simulink model "AllProject"  (R2018b)
settings: Solver=VariableStepAuto  StartTime=0.0  StopTime=10  RelTol=1e-3
values from neighbouring files (symbols this model uses):
  alphaTemperature = (65.5/180)*pi    (= 1.14319066006)    [project.m]
  Ik = 0.38    [project.m]
  Iw = 0.26    [project.m]
  Iz = 1.08    [project.m]
  rk = 0.22    [project.m]
  rw = 0.1    [project.m]
settings Model: Creator=AmirHosein Rostami  LastModifiedBy=AmirHosein Rostami

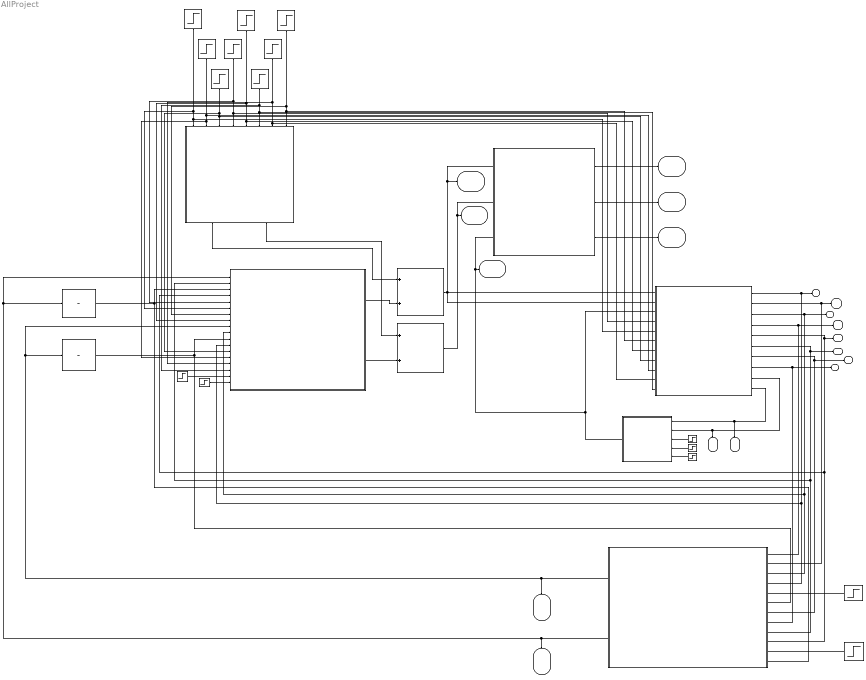
== system AllProject ==
  Add : Sum
  Add1 : Sum
  BallSegway : Subsystem
  Integrator : Integrator
  Integrator1 : Integrator
  LQR : MATLAB Function  TreatAsAtomicUnit=on
  PIController_KP_KI : MATLAB Function  TreatAsAtomicUnit=on
  PIDController : MATLAB Function  TreatAsAtomicUnit=on
  Step : Step  SampleTime=0
  Step1 : Step  SampleTime=0
  Step{10..13} (4 alike) : Step  After=1000  SampleTime=0
  Step2 : Step  After=pi/6  SampleTime=0
  Step{7..9,21} (4 alike) : Step  After=100  SampleTime=0
  Step3 : Step  Time=0  After=0  SampleTime=0
  Step4 : Step  Time=0  After=0  SampleTime=0
  Step5 : Step  After=2.5  SampleTime=0
  Step6 : Step  After=0.2  SampleTime=0
  frictions : MATLAB Function  TreatAsAtomicUnit=on
  torqueConversion2 : MATLAB Function  TreatAsAtomicUnit=on
  TauX : Outport
  TauY : Outport  Port=2
  TauZ : Outport  Port=3
  thetaX : Outport  Port=4
  thetaY : Outport  Port=5
  Vx : Outport  Port=6
  Vy : Outport  Port=7
  xk : Outport  Port=8
  xkDot : Outport  Port=9
  thetaYDot : Outport  Port=10
  yk : Outport  Port=11
  ykDot : Outport  Port=12
  thetaXDot : Outport  Port=13
  Tau1 : Outport  Port=14
  Tau2 : Outport  Port=15
  Tau3 : Outport  Port=16
  thetaZ : Outport  Port=17
  thetaZDot : Outport  Port=18
  wires:
  BallSegway/7("thetaXDot ") -> thetaXDot/1, LQR/7(thetaXDot)
  frictions/1(Uxf) -> Add/1
  frictions/2(Uyf) -> Add1/1
  LQR/1(vx) -> Vx/1, PIController_KP_KI/9(vx), Integrator1/1
  LQR/2(vy) -> Vy/1, PIController_KP_KI/1(vy), Integrator/1
  BallSegway/4("thetaYDot ") -> LQR/1(thetaYDot), thetaYDot/1
  BallSegway/2(thetaY) -> LQR/2(thetaY), thetaY/1
  Integrator/1 -> LQR/12(x5r), PIController_KP_KI/3(x5r)
  Integrator1/1 -> LQR/6(x5p), PIController_KP_KI/11(x5p)
  Add/1 -> BallSegway/2(Taux), TauX/1, torqueConversion2/1(tauX), BallSegway/1(TauY)
  PIDController/1(TauZ) -> BallSegway/3(TauZ), TauZ/1, torqueConversion2/3(tauZ)  "TauZ"
  BallSegway/9(Xz) -> PIDController/2(theta), thetaZ/1  "thetaZ"
  BallSegway/10(XzDot) -> PIDController/1(thetaZDot), thetaZDot/1  "thetaZDot"
  BallSegway/8("thetaX ") -> LQR/8(thetaX), thetaX/1
  Step/1 -> PIDController/3(kdz)
  Step1/1 -> PIDController/4(kpz)
  Step2/1 -> PIDController/5(thetaZDestination)
  BallSegway/1(xk) -> xk/1, LQR/4(xk), PIController_KP_KI/12(xk)
  BallSegway/5(yk) -> yk/1, LQR/10(yk), PIController_KP_KI/4(yk)
  BallSegway/3(xkDot) -> LQR/3(xkDot), PIController_KP_KI/10(xkDot), xkDot/1
  BallSegway/6(ykDot) -> ykDot/1, LQR/9(ykDot), PIController_KP_KI/2(ykDot)
  Step5/1 -> PIController_KP_KI/17(Wn)
  Step6/1 -> PIController_KP_KI/18(kessi)
  Step7/1 -> BallSegway/9(bry), PIController_KP_KI/14(bry), frictions/2(bry)
  Step8/1 -> PIController_KP_KI/13(bx), BallSegway/8(bx), frictions/3(bx)
  Step9/1 -> BallSegway/4(by), frictions/4(by), PIController_KP_KI/5(by)
  Step10/1 -> PIController_KP_KI/8(drx), BallSegway/7(drx), frictions/5(drx)
  Step11/1 -> PIController_KP_KI/16(dry), BallSegway/11(dry), frictions/6(dry)
  Step12/1 -> PIController_KP_KI/15(dx), BallSegway/10(dx), frictions/7(dx)
  Step13/1 -> PIController_KP_KI/7(dy), BallSegway/6(dy), frictions/8(dy)
  Step21/1 -> PIController_KP_KI/6(brx), BallSegway/5(brx), frictions/1(brx)
  PIController_KP_KI/1(uPIx) -> Add/2
  PIController_KP_KI/2(uPIy) -> Add1/2
  torqueConversion2/1(tau1) -> Tau1/1
  torqueConversion2/2(tau2) -> Tau2/1
  torqueConversion2/3(tau3) -> Tau3/1
  Add1/1 -> TauY/1, torqueConversion2/2(tauY)
  Step3/1 -> LQR/11(ykd)
  Step4/1 -> LQR/5(xkd)

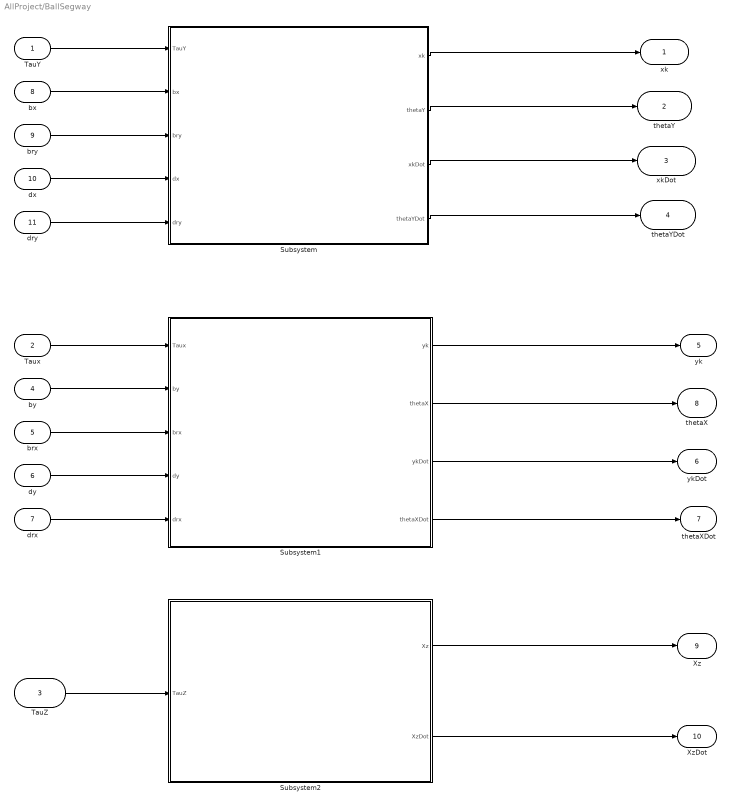
== system AllProject/BallSegway ==
  TauY : Inport
  Taux : Inport  Port=2
  TauZ : Inport  Port=3
  by : Inport  Port=4
  brx : Inport  Port=5
  dy : Inport  Port=6
  drx : Inport  Port=7
  bx : Inport  Port=8
  bry : Inport  Port=9
  dx : Inport  Port=10
  dry : Inport  Port=11
  Subsystem : Subsystem
  Subsystem1 : Subsystem
  Subsystem2 : Subsystem
  xk : Outport
  thetaY : Outport  Port=2
  xkDot : Outport  Port=3
  "thetaYDot " : Outport  Port=4
  yk : Outport  Port=5
  ykDot : Outport  Port=6
  "thetaXDot " : Outport  Port=7
  "thetaX " : Outport  Port=8
  Xz : Outport  Port=9
  XzDot : Outport  Port=10
  wires:
  Subsystem2/1(Xz) -> Xz/1
  TauZ/1 -> Subsystem2/1(TauZ)
  Subsystem2/2(XzDot) -> XzDot/1
  Subsystem/3(xkDot) -> xkDot/1
  Subsystem/4("thetaYDot ") -> "thetaYDot "/1
  Subsystem/1(xk) -> xk/1
  TauY/1 -> Subsystem/1(TauY)
  Taux/1 -> Subsystem1/1(Taux)
  Subsystem1/1(yk) -> yk/1
  Subsystem/2(thetaY) -> thetaY/1
  Subsystem1/4("thetaXDot ") -> "thetaXDot "/1
  Subsystem1/2(thetaX) -> "thetaX "/1
  Subsystem1/3(ykDot) -> ykDot/1
  by/1 -> Subsystem1/2(by)
  brx/1 -> Subsystem1/3(brx)
  dy/1 -> Subsystem1/4(dy)
  drx/1 -> Subsystem1/5(drx)
  bx/1 -> Subsystem/2(bx)
  bry/1 -> Subsystem/3(bry)
  dx/1 -> Subsystem/4(dx)
  dry/1 -> Subsystem/5(dry)

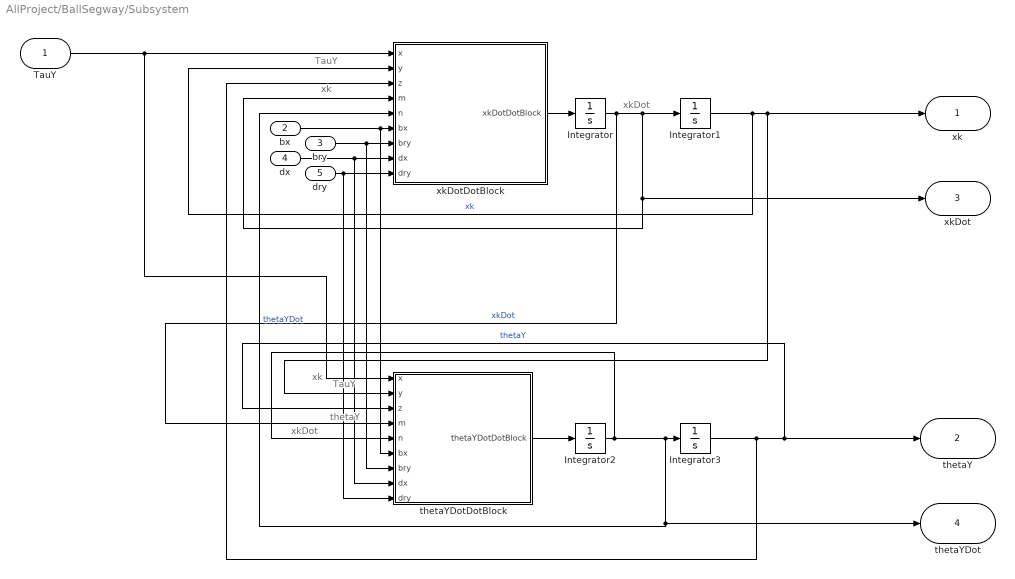
== system AllProject/BallSegway/Subsystem ==
  note: xk
  note: TauY
  note: TauY
  note: xkDot
  note: xk
  note: xkDot
  note: thetaY
  TauY : Inport
  bx : Inport  Port=2
  bry : Inport  Port=3
  dx : Inport  Port=4
  dry : Inport  Port=5
  Integrator : Integrator
  Integrator1 : Integrator
  Integrator2 : Integrator
  Integrator3 : Integrator  InitialCondition=(0.1/180)*pi
  thetaYDotDotBlock : MATLAB Function  TreatAsAtomicUnit=on
  xkDotDotBlock : MATLAB Function  TreatAsAtomicUnit=on
  xk : Outport
  thetaY : Outport  Port=2
  xkDot : Outport  Port=3
  "thetaYDot " : Outport  Port=4
  wires:
  Integrator/1 -> thetaYDotDotBlock/4(m), xkDotDotBlock/4(m), xkDot/1, Integrator1/1  "xkDot"
  Integrator1/1 -> xkDotDotBlock/2(y), thetaYDotDotBlock/2(y), xk/1  "xk"
  Integrator2/1 -> thetaYDotDotBlock/5(n), xkDotDotBlock/5(n), "thetaYDot "/1, Integrator3/1  "thetaYDot"
  xkDotDotBlock/1(xkDotDotBlock) -> Integrator/1
  Integrator3/1 -> xkDotDotBlock/3(z), thetaYDotDotBlock/3(z), thetaY/1  "thetaY"
  TauY/1 -> thetaYDotDotBlock/1(x), xkDotDotBlock/1(x)
  thetaYDotDotBlock/1(thetaYDotDotBlock) -> Integrator2/1
  bx/1 -> thetaYDotDotBlock/6(bx), xkDotDotBlock/6(bx)
  bry/1 -> xkDotDotBlock/7(bry), thetaYDotDotBlock/7(bry)
  dx/1 -> xkDotDotBlock/8(dx), thetaYDotDotBlock/8(dx)
  dry/1 -> xkDotDotBlock/9(dry), thetaYDotDotBlock/9(dry)

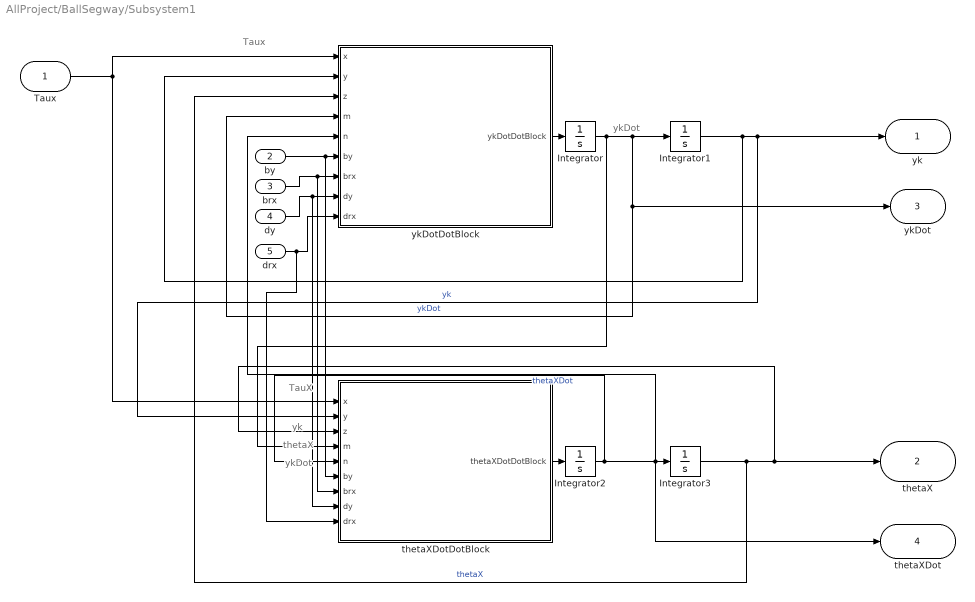
== system AllProject/BallSegway/Subsystem1 ==
  note: yk
  note: Taux
  note: thetaX
  note: ykDot
  note: TauX
  note: ykDot
  Taux : Inport
  by : Inport  Port=2
  brx : Inport  Port=3
  dy : Inport  Port=4
  drx : Inport  Port=5
  Integrator : Integrator
  Integrator1 : Integrator
  Integrator2 : Integrator
  Integrator3 : Integrator  InitialCondition=(0.1/180)*pi
  thetaXDotDotBlock : MATLAB Function  TreatAsAtomicUnit=on
  ykDotDotBlock : MATLAB Function  TreatAsAtomicUnit=on
  yk : Outport
  thetaX : Outport  Port=2
  ykDot : Outport  Port=3
  "thetaXDot " : Outport  Port=4
  wires:
  Integrator2/1 -> thetaXDotDotBlock/5(n), "thetaXDot "/1, ykDotDotBlock/5(n), Integrator3/1  "thetaXDot"
  Taux/1 -> ykDotDotBlock/1(x), thetaXDotDotBlock/1(x)
  Integrator/1 -> thetaXDotDotBlock/4(m), ykDotDotBlock/4(m), ykDot/1, Integrator1/1  "ykDot"
  Integrator1/1 -> ykDotDotBlock/2(y), thetaXDotDotBlock/2(y), yk/1  "yk"
  thetaXDotDotBlock/1(thetaXDotDotBlock) -> Integrator2/1
  Integrator3/1 -> ykDotDotBlock/3(z), thetaXDotDotBlock/3(z), thetaX/1  "thetaX"
  ykDotDotBlock/1(ykDotDotBlock) -> Integrator/1
  by/1 -> ykDotDotBlock/6(by), thetaXDotDotBlock/6(by)
  brx/1 -> ykDotDotBlock/7(brx), thetaXDotDotBlock/7(brx)
  dy/1 -> ykDotDotBlock/8(dy), thetaXDotDotBlock/8(dy)
  drx/1 -> ykDotDotBlock/9(drx), thetaXDotDotBlock/9(drx)

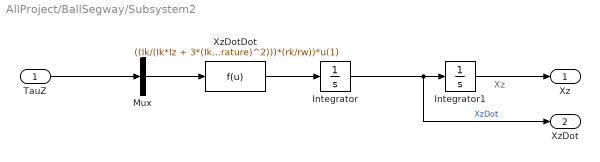
== system AllProject/BallSegway/Subsystem2 ==
  note: Xz
  TauZ : Inport
  Integrator : Integrator  ContinuousStateAttributes='XzDot'
  Integrator1 : Integrator  ContinuousStateAttributes='Xz'
  Mux : Mux  Inputs=1
  XzDotDot : Fcn  Expr=((Ik/(Ik*Iz + 3*(Ik+Iz)*Iw*((rk^2)/(rw^2))*(sin(alphaTemperature)^2)))*(rk/rw))*u(1)
  Xz : Outport
  XzDot : Outport  Port=2
  wires:
  Mux/1 -> XzDotDot/1
  TauZ/1 -> Mux/1
  Integrator1/1 -> Xz/1
  XzDotDot/1 -> Integrator/1
  Integrator/1 -> XzDot/1, Integrator1/1  "XzDot"

== matlab function AllProject/BallSegway/Subsystem1/thetaXDotDotBlock ==
  data: x input; thetaXDotDotBlock output; y input; z input; m input; n input; by input; brx input; dy input; drx input
function thetaXDotDotBlock = thetaXDotDotBlock(x,y,z,m,n,by,brx,dy,drx)
%#codegen

%    This function was generated by the Symbolic Math Toolbox version 8.2.
%    27-Jan-2020 23:39:11

t2 = cos(z);
t3 = sin(z);
t4 = t2.*(3.0./4.0e1);
t5 = t2.^2;
t9 = t5.*(1.3e1./2.0e1);
t6 = t4-t9+1.1e1./5.0;
t7 = 1.0./t6;
t8 = z.^2;
t10 = sign(m);
thetaXDotDotBlock = t7.*(dy.*t10.*1.5e-3-(drx.*sign(n))./1.0e1)-(by.*m.*(-1.5e-3)+(brx.*n)./1.0e1+(by.*m.*t2)./4.0e1)./(t4-cos(t8).*(1.3e1./2.0e1)+1.1e1./5.0)+t7.*(t3.*(2.51e2./1.0e1)-t8.*sin(z.*2.0).*(8.0./2.5e1)+n.^2.*t3.*(3.7e1./1.0e3))+t7.*x.*(t2./4.0+2.1e1./1.0e2)+(dy.*t2.*t7.*t10)./4.0e1;

== matlab function AllProject/BallSegway/Subsystem/thetaYDotDotBlock ==
  data: x input; thetaYDotDotBlock output; y input; z input; m input; n input; bx input; bry input; dx input; dry input
function thetaYDotDotBlock = thetaYDotDotBlock(x,y,z,m,n,bx,bry,dx,dry)
%#codegen

%    This function was generated by the Symbolic Math Toolbox version 8.2.
%    28-Jan-2020 00:14:21

t2 = cos(z);
t3 = sin(z);
t4 = t2.*(3.0./4.0e1);
t5 = t2.^2;
t9 = t5.*(1.3e1./2.0e1);
t6 = t4-t9+1.1e1./5.0;
t7 = 1.0./t6;
t8 = z.^2;
t10 = sign(m);
thetaYDotDotBlock = -t7.*(dx.*t10.*1.5e-3+(dry.*sign(n))./1.0e1)-(bx.*m.*1.5e-3+(bry.*n)./1.0e1-(bx.*m.*t2)./4.0e1)./(t4-cos(t8).*(1.3e1./2.0e1)+1.1e1./5.0)+t7.*(t3.*(2.51e2./1.0e1)-t8.*sin(z.*2.0).*(8.0./2.5e1)+n.^2.*t3.*(3.7e1./1.0e3))+t7.*x.*(t2./4.0+2.1e1./1.0e2)+(dx.*t2.*t7.*t10)./4.0e1;

== matlab function AllProject/frictions ==
  data: Uxf output; Uyf output; brx input; bry input; bx input; by input; drx input; dry input; dx input; dy input
function [Uxf,Uyf] = frictions(brx,bry,bx,by,drx,dry,dx,dy)
%#codegen

%    This function was generated by the Symbolic Math Toolbox version 8.2.
%    28-Jan-2020 01:09:16

Uxf = brx.*9.074074074069469e-8+by.*8.333333333333526e-8+drx.*9.074074074065839e-2+dy.*8.333333333330192e-2-2.285370370367702e-5;
if nargout > 1
    Uyf = bry.*9.074074074065839e-8-bx.*8.148148148145077e-8-dry.*1.018518518517653e-1-dx.*8.148148148145077e-2-2.285370370367706e-5;
end

== matlab function AllProject/PIDController ==
  data: thetaZDot input; TauZ output; theta input; kdz input; kpz input; thetaZDestination input
function TauZ = PIDController(thetaZDot,theta,kdz,kpz,thetaZDestination)
%#codegen

%    This function was generated by the Symbolic Math Toolbox version 8.2.
%    26-Jan-2020 14:57:10

TauZ = kdz.*thetaZDot+kpz.*(theta-thetaZDestination);

== matlab function AllProject/PIController_KP_KI ==
  data: vy input; uPIx output; ykDot input; x5r input; yk input; by input; brx input; dy input; drx input; vx input; xkDot input; x5p input; xk input; bx input; bry input; dx input; dry input; Wn input; kessi input; uPIy output
function [uPIx,uPIy] = PIController_KP_KI(vy,ykDot,x5r,yk,by,brx,dy,drx,vx,xkDot,x5p,xk,bx,bry,dx,dry,Wn,kessi)
%#codegen

%    This function was generated by the Symbolic Math Toolbox version 8.2.
%    28-Jan-2020 01:08:50

t2 = Wn.^2;
uPIx = t2.*(x5r-yk).*(3.25e2./5.4e1)+Wn.*kessi.*(vy-ykDot).*(3.25e2./2.7e1);
if nargout > 1
    t3 = cos(1.0./1.0e3);
    t4 = t3.*(3.0./5.0e1);
    t5 = t4+2.1e1./1.0e2;
    t6 = 1.0./t5;
    t7 = t3.*(3.0./4.0e1);
    t8 = t3.^2;
    t9 = t7-t8.*(1.3e1./2.0e1)+1.1e1./5.0;
    uPIy = -t2.*t6.*t9.*(x5p-xk)-Wn.*kessi.*t6.*t9.*(vx-xkDot).*2.0;
end

== matlab function AllProject/LQR ==
  data: thetaYDot input; vx output; thetaY input; xkDot input; xk input; xkd input; x5p input; thetaXDot input; thetaX input; ykDot input; yk input; ykd input; x5r input; vy output
function [vx,vy] = LQR(thetaYDot,thetaY,xkDot,xk,xkd,x5p,thetaXDot,thetaX,ykDot,yk,ykd,x5r)
%#codegen

%    This function was generated by the Symbolic Math Toolbox version 8.2.
%    26-Jan-2020 21:37:42

vx = thetaY.*(-4.01e2./1.0e2)+thetaYDot.*(3.27e2./1.0e2)-x5p.*(1.43e2./2.5e1)-xk.*(4.27e2./5.0e1)-xkDot.*2.907e1+xkd.*(4.27e2./5.0e1);
if nargout > 1
    vy = thetaX.*(8.9e1./2.0e1)+thetaXDot.*(3.49e2./5.0e1)-x5r.*(5.11e2./1.0e2)-yk.*(6.09e2./1.0e2)-ykDot.*(5.22e2./2.5e1)+ykd.*(6.09e2./1.0e2);
end

== matlab function AllProject/torqueConversion2 ==
  data: tauX input; tau1 output; tauY input; tauZ input; tau2 output; tau3 output
function [tau1,tau2,tau3] = torqueConversion(tauX,tauY,tauZ)
%#codegen

%    This function was generated by the Symbolic Math Toolbox version 8.2.
%    24-Jan-2020 16:45:38

t2 = pi.*(1.33e2./3.6e2);
t3 = cos(t2);
t4 = 1.0./t3;
t5 = sin(t2);
t6 = 1.0./t5;
t7 = (t6.*tauZ)./3.0;
tau1 = t7+t4.*tauX.*(2.0./3.0);
if nargout > 1
    t8 = sqrt(3.0);
    t9 = (t4.*t8.*tauY)./3.0;
    tau2 = t7+t9-(t4.*tauX)./3.0;
end
if nargout > 2
    tau3 = t7-t9-(t4.*tauX)./3.0;
end

== matlab function AllProject/BallSegway/Subsystem1/ykDotDotBlock ==
  data: x input; ykDotDotBlock output; y input; z input; m input; n input; by input; brx input; dy input; drx input
function ykDotDotBlock = ykDotDotBlock(x,y,z,m,n,by,brx,dy,drx)
%#codegen

%    This function was generated by the Symbolic Math Toolbox version 8.2.
%    29-Jan-2020 03:11:04

t2 = cos(z);
t3 = sin(z);
t4 = t2.*(3.0./4.0e1);
t5 = t2.^2;
t8 = t5.*(1.3e1./2.0e1);
t6 = t4-t8+1.1e1./5.0;
t7 = 1.0./t6;
t9 = sign(n);
ykDotDotBlock = (t7.*(drx.*t9.*(3.0./1.0e2)-dy.*sign(m).*(9.0./2.0e1)))./2.0e1-(t7.*(by.*m.*(9.0./2.0e1)-brx.*n.*(3.0./1.0e2)+brx.*n.*t2.*(1.3e1./2.5e1)))./2.0e1-(t7.*(t3.*(7.59e2./1.0e2)-sin(z.*2.0).*(1.31e2./2.0)+n.^2.*t3.*(2.3e1./2.0)))./2.0e1+t7.*x.*(t2.*(3.0./5.0e1)+2.1e1./1.0e2)-drx.*t2.*t7.*t9.*(1.3e1./5.0e2);

== matlab function AllProject/BallSegway/Subsystem/xkDotDotBlock ==
  data: x input; xkDotDotBlock output; y input; z input; m input; n input; bx input; bry input; dx input; dry input
function xkDotDotBlock = xkDotDotBlock(x,y,z,m,n,bx,bry,dx,dry)
%#codegen

%    This function was generated by the Symbolic Math Toolbox version 8.2.
%    28-Jan-2020 00:14:20

t2 = cos(z);
t3 = sin(z);
t4 = t2.*(3.0./4.0e1);
t5 = t2.^2;
t8 = t5.*(1.3e1./2.0e1);
t6 = t4-t8+1.1e1./5.0;
t7 = 1.0./t6;
t9 = sign(n);
xkDotDotBlock = t7.*(dry.*t9.*(3.0./1.0e2)+dx.*sign(m).*(1.1e1./2.5e1)).*(-1.0./2.0e1)-(t7.*(bx.*m.*(1.1e1./2.5e1)+bry.*n.*(3.0./1.0e2)-bry.*n.*t2.*(1.3e1./2.5e1)))./2.0e1+(t7.*(t3.*(7.59e2./1.0e2)-sin(z.*2.0).*(1.31e2./2.0)+n.^2.*t3.*(1.13e2./1.0e1)))./2.0e1-t7.*x.*(t2.*(3.0./5.0e1)+2.1e1./1.0e2)-dry.*t2.*t7.*t9.*(1.3e1./5.0e2);
